simulink model "water_4hopper_VDF"  (Simulink 8.0)
settings: Solver=ode23  StartTime=0.0  StopTime=30  RelTol=1e-3
values from neighbouring files (symbols this model uses):
  alpha = 30    [SimParam_4VDF.m]
  Amp = leg_length    (= 0.0249)    [SimParam_4VDF.m]
  b_water = 0.5*C_d*S1*density    (= 0.405708731037)    [SimParam_4VDF.m]
  C_d = 0.703    [SimParam.m]    (also in SimParam_4VDF.m)
  density = 1000    [SimParam.m]    (also in SimParam_4VDF.m)
  frame_inertia = diag([Ix,Iy,Iz])    [SimParam.m]    (also in SimParam_4VDF.m)
  Fratio = 1/16    (= 0.0625)    [SimParam_4VDF.m]
  freq = 20    [SimParam.m]    (also in SimParam_4VDF.m = 60)
  g = 9.81    [SimParam.m]    (also in SimParam_4VDF.m)
  k_water = C_d*S1*density*g    (= 7.96000530294)    [SimParam_4VDF.m]
  leg_length = 0.06    [SimParam.m]    (also in SimParam_4VDF.m = 0.0249)
  Lx = frame_width/2*[-1 -1 1 1]'    [SimParam_4VDF.m]
  Lxmat = frame_width/2*[-1 0 0 0 ; 0 -1 0 0 ; 0 0 1 0 ; 0 0 0 1]    [SimParam_4VDF.m]
  Lz = frame_length/2*[-1 1 1 -1]'    [SimParam_4VDF.m]
  Lzmat = frame_length/2*[-1 0 0 0 ; 0 1 0 0 ; 0 0 1 0 ; 0 0 0 -1]    [SimParam_4VDF.m]
  mass = 0.1    [SimParam.m]    (also in SimParam_4VDF.m)
  mass_matrix = [mass 0 0; 0 Ix 0 ; 0 0 Iz]    [SimParam_4VDF.m]
  omega_0 = freq*ones(8,1)    [SimParam_4VDF.m]
  S1 = pi*r1^2    (= 0.00125663706144)    [SimParam.m]    (also in SimParam_4VDF.m = 0.00115422114093)
  S2 = pi*r2^2    (= 7.85398163397e-05)    [SimParam.m]    (also in SimParam_4VDF.m = 7.21388213081e-05)
  tau = 0.005    [SimParam_4VDF.m]
  wave = eps    [SimParam_4VDF.m]
  wavefreq = .5    (= 0.5)    [SimParam_4VDF.m]
undefined symbols (not defined in the file): amp, cw_FL_HL, cw_FR_FL, cw_FR_HR, cw_HR_HL, Filter_Coef, FL_HL_lag, FR_FL_lag, FR_HR_lag, HR_HL_lag, K_d, K_i, K_p, y_0
libraries: mblibv1 x34, dspstat3 x6, dspinverses x1
(part 2 of 2)

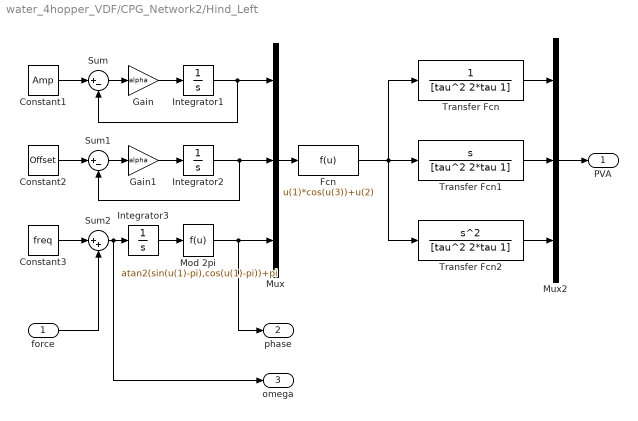
== system water_4hopper_VDF/CPG_Network2/Hind_Left ==
  force : Inport
  Constant1 : Constant  Value=Amp
  Constant2 : Constant  Value=Offset
  Constant3 : Constant  Value=freq
  Fcn : Fcn  Expr=u(1)*cos(u(3))+u(2)
  Gain : Gain  Gain=alpha
  Gain1 : Gain  Gain=alpha
  Integrator1 : Integrator
  Integrator2 : Integrator
  Integrator3 : Integrator  InitialCondition=init_phi + 0.01*rand
  Mod 2pi : Fcn  Expr=atan2(sin(u(1)-pi),cos(u(1)-pi))+pi
  Mux : Mux  Inputs=3
  Mux2 : Mux  Inputs=3
  Sum : Sum  Inputs=|+-
  Sum1 : Sum  Inputs=|+-
  Sum2 : Sum  Inputs=|++
  Transfer Fcn : TransferFcn  Denominator=[tau^2 2*tau 1]
  Transfer Fcn1 : TransferFcn  Numerator=[1 0]  Denominator=[tau^2 2*tau 1]
  Transfer Fcn2 : TransferFcn  Numerator=[1 0 0]  Denominator=[tau^2 2*tau 1]
  PVA : Outport
  phase : Outport  Port=2
  omega : Outport  Port=3
  wires:
  Sum/1 -> Gain/1
  Integrator1/1 -> Sum/2, Mux/1
  Constant1/1 -> Sum/1
  Gain/1 -> Integrator1/1
  Sum1/1 -> Gain1/1
  Integrator2/1 -> Sum1/2, Mux/2
  Constant2/1 -> Sum1/1
  Gain1/1 -> Integrator2/1
  Mux/1 -> Fcn/1
  Mod 2pi/1 -> phase/1, Mux/3
  Integrator3/1 -> Mod 2pi/1
  Constant3/1 -> Sum2/1
  Sum2/1 -> omega/1, Integrator3/1
  force/1 -> Sum2/2
  Transfer Fcn2/1 -> Mux2/3
  Transfer Fcn/1 -> Mux2/1
  Transfer Fcn1/1 -> Mux2/2
  Fcn/1 -> Transfer Fcn2/1, Transfer Fcn/1, Transfer Fcn1/1
  Mux2/1 -> PVA/1

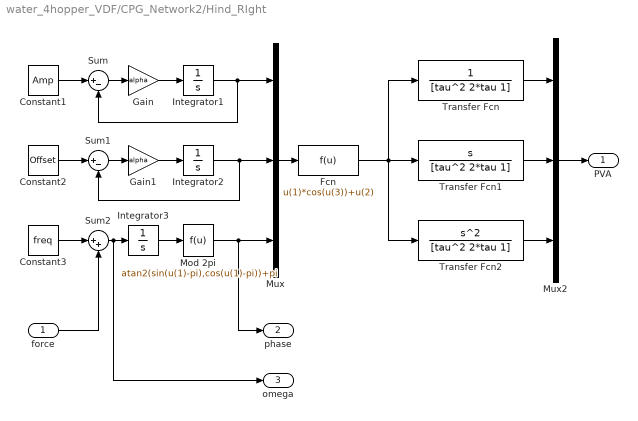
== system water_4hopper_VDF/CPG_Network2/Hind_RIght ==
  force : Inport
  Constant1 : Constant  Value=Amp
  Constant2 : Constant  Value=Offset
  Constant3 : Constant  Value=freq
  Fcn : Fcn  Expr=u(1)*cos(u(3))+u(2)
  Gain : Gain  Gain=alpha
  Gain1 : Gain  Gain=alpha
  Integrator1 : Integrator
  Integrator2 : Integrator
  Integrator3 : Integrator  InitialCondition=init_phi + 0.01*rand
  Mod 2pi : Fcn  Expr=atan2(sin(u(1)-pi),cos(u(1)-pi))+pi
  Mux : Mux  Inputs=3
  Mux2 : Mux  Inputs=3
  Sum : Sum  Inputs=|+-
  Sum1 : Sum  Inputs=|+-
  Sum2 : Sum  Inputs=|++
  Transfer Fcn : TransferFcn  Denominator=[tau^2 2*tau 1]
  Transfer Fcn1 : TransferFcn  Numerator=[1 0]  Denominator=[tau^2 2*tau 1]
  Transfer Fcn2 : TransferFcn  Numerator=[1 0 0]  Denominator=[tau^2 2*tau 1]
  PVA : Outport
  phase : Outport  Port=2
  omega : Outport  Port=3
  wires:
  Sum/1 -> Gain/1
  Integrator1/1 -> Sum/2, Mux/1
  Constant1/1 -> Sum/1
  Gain/1 -> Integrator1/1
  Sum1/1 -> Gain1/1
  Integrator2/1 -> Sum1/2, Mux/2
  Constant2/1 -> Sum1/1
  Gain1/1 -> Integrator2/1
  Mux/1 -> Fcn/1
  Mod 2pi/1 -> phase/1, Mux/3
  Integrator3/1 -> Mod 2pi/1
  Constant3/1 -> Sum2/1
  Sum2/1 -> omega/1, Integrator3/1
  force/1 -> Sum2/2
  Transfer Fcn2/1 -> Mux2/3
  Transfer Fcn/1 -> Mux2/1
  Transfer Fcn1/1 -> Mux2/2
  Fcn/1 -> Transfer Fcn2/1, Transfer Fcn/1, Transfer Fcn1/1
  Mux2/1 -> PVA/1

== system water_4hopper_VDF/CPG_Network2/split FL ==
  w_pos : Inport
  PVA : Inport  Port=2
  w_neg : Inport  Port=3
  Product : Product  RndMeth=Zero
  Product1 : Product  RndMeth=Zero
  Sum2 : Sum  Inputs=|++
  enable : Subsystem
  sel : Selector  InputPortWidth=3  IndexOptions=Index vector (dialog)  Indices=[2]  OutputSizes=1
  Force : Outport
  wires:
  Product/1 -> Sum2/1
  w_pos/1 -> Product/1
  w_neg/1 -> Product1/1
  Product1/1 -> Sum2/2
  PVA/1 -> sel/1
  enable/1(pos) -> Product/2
  enable/2(neg) -> Product1/2
  Sum2/1 -> Force/1
  sel/1 -> enable/1(in)

== system water_4hopper_VDF/CPG_Network2/split FL1 ==
  w_pos : Inport
  PVA : Inport  Port=2
  w_neg : Inport  Port=3
  Product : Product  RndMeth=Zero
  Product1 : Product  RndMeth=Zero
  Sum2 : Sum  Inputs=|++
  enable : Subsystem
  sel : Selector  InputPortWidth=3  IndexOptions=Index vector (dialog)  Indices=[2]  OutputSizes=1
  Force : Outport
  wires:
  sel/1 -> enable/1(in)
  Sum2/1 -> Force/1
  enable/2(neg) -> Product1/2
  enable/1(pos) -> Product/2
  PVA/1 -> sel/1
  Product1/1 -> Sum2/2
  w_neg/1 -> Product1/1
  w_pos/1 -> Product/1
  Product/1 -> Sum2/1

== system water_4hopper_VDF/CPG_Network2/split FL2 ==
  w_pos : Inport
  PVA : Inport  Port=2
  w_neg : Inport  Port=3
  Product : Product  RndMeth=Zero
  Product1 : Product  RndMeth=Zero
  Sum2 : Sum  Inputs=|++
  enable : Subsystem
  sel : Selector  InputPortWidth=3  IndexOptions=Index vector (dialog)  Indices=[2]  OutputSizes=1
  Force : Outport
  wires:
  Product/1 -> Sum2/1
  w_pos/1 -> Product/1
  w_neg/1 -> Product1/1
  Product1/1 -> Sum2/2
  PVA/1 -> sel/1
  enable/1(pos) -> Product/2
  enable/2(neg) -> Product1/2
  Sum2/1 -> Force/1
  sel/1 -> enable/1(in)

== system water_4hopper_VDF/CPG_Network2/split FL3 ==
  w_pos : Inport
  PVA : Inport  Port=2
  w_neg : Inport  Port=3
  Product : Product  RndMeth=Zero
  Product1 : Product  RndMeth=Zero
  Sum2 : Sum  Inputs=|++
  enable : Subsystem
  sel : Selector  InputPortWidth=3  IndexOptions=Index vector (dialog)  Indices=[2]  OutputSizes=1
  Force : Outport
  wires:
  Product/1 -> Sum2/1
  w_pos/1 -> Product/1
  w_neg/1 -> Product1/1
  Product1/1 -> Sum2/2
  PVA/1 -> sel/1
  enable/1(pos) -> Product/2
  enable/2(neg) -> Product1/2
  Sum2/1 -> Force/1
  sel/1 -> enable/1(in)

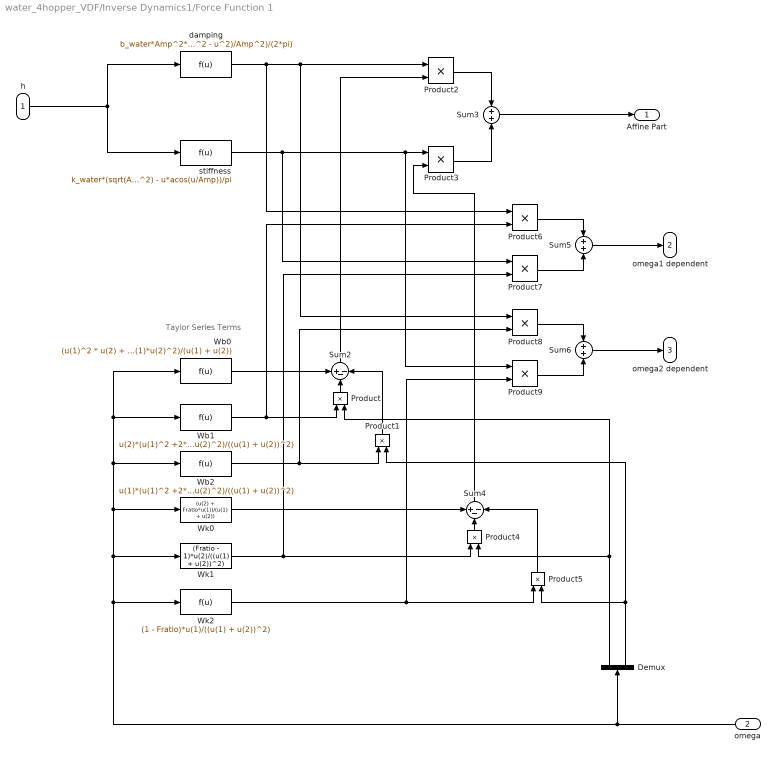
== system water_4hopper_VDF/Inverse Dynamics1/Force Function 1 ==
  note: Taylor Series Terms
  h : Inport
  omega : Inport  Port=2
  Demux : Demux  Outputs=2
  Product{,1..9} (10 alike) : Product  RndMeth=Zero
  Sum2 : Sum  Inputs=+--
  Sum3 : Sum  Inputs=+|+
  Sum4 : Sum  Inputs=+--
  Sum5 : Sum  Inputs=+|+
  Sum6 : Sum  Inputs=+|+
  Wb0 : Fcn  Expr=(u(1)^2 * u(2) + Fratio*u(1)*u(2)^2)/(u(1) + u(2))
  Wb1 : Fcn  Expr=u(2)*(u(1)^2 +2*u(1)*u(2) + Fratio*u(2)^2)/((u(1) + u(2))^2)
  Wb2 : Fcn  Expr=u(1)*(u(1)^2 +2*Fratio*u(1)*u(2) + Fratio*u(2)^2)/((u(1) + u(2))^2)
  Wk0 : Fcn  Expr=(u(2) + Fratio*u(1))/(u(1) + u(2))
  Wk1 : Fcn  Expr=(Fratio - 1)*u(2)/((u(1) + u(2))^2)
  Wk2 : Fcn  Expr=(1 - Fratio)*u(1)/((u(1) + u(2))^2)
  damping : Fcn  Expr=b_water*Amp^2*(acos(u/Amp) - u*sqrt(Amp^2 - u^2)/Amp^2)/(2*pi)
  stiffness : Fcn  Expr=k_water*(sqrt(Amp^2 - u^2) - u*acos(u/Amp))/pi
  Affine Part : Outport
  omega1 dependent : Outport  Port=2
  omega2 dependent : Outport  Port=3
  wires:
  Product2/1 -> Sum3/1
  Product9/1 -> Sum6/2
  Wb1/1 -> Product6/2, Product/1
  Product4/1 -> Sum4/2
  Wb0/1 -> Sum2/1
  Product7/1 -> Sum5/2
  Wk1/1 -> Product7/2, Product4/1
  Wk0/1 -> Sum4/1
  Product6/1 -> Sum5/1
  Wb2/1 -> Product8/2, Product1/1
  Product/1 -> Sum2/2
  Sum3/1 -> Affine Part/1
  Product1/1 -> Sum2/3
  stiffness/1 -> Product7/1, Product9/1, Product3/1
  Wk2/1 -> Product5/1, Product9/2
  damping/1 -> Product6/1, Product8/1, Product2/1
  Product5/1 -> Sum4/3
  Product3/1 -> Sum3/2
  Sum5/1 -> omega1 dependent/1
  Sum4/1 -> Product3/2
  omega/1 -> Wb0/1, Wb1/1, Wb2/1, Wk0/1, Wk1/1, Wk2/1, Demux/1
  Sum2/1 -> Product2/2
  Product8/1 -> Sum6/1
  Sum6/1 -> omega2 dependent/1
  Demux/1 -> Product4/2, Product/2
  Demux/2 -> Product5/2, Product1/2
  h/1 -> stiffness/1, damping/1

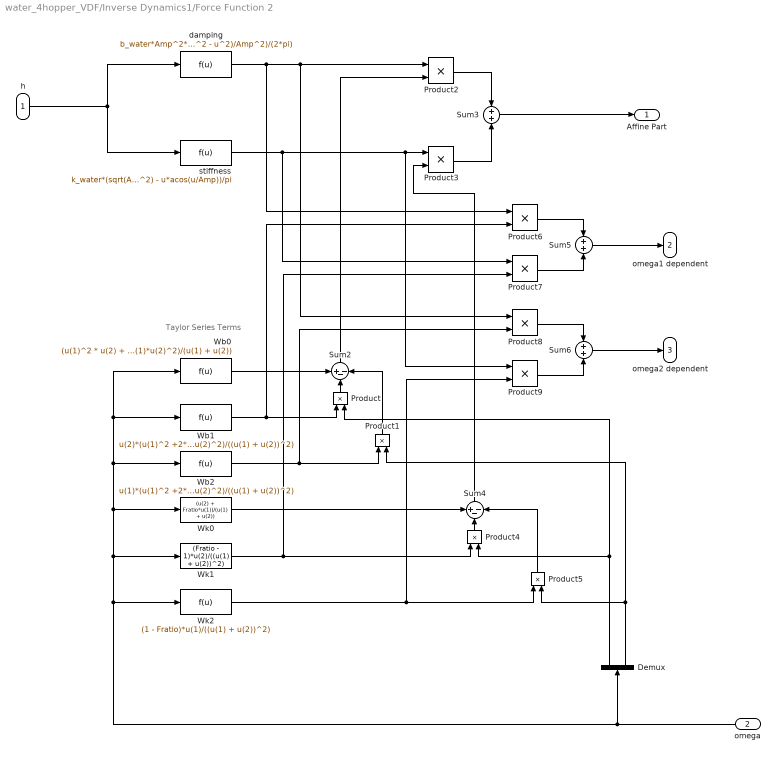
== system water_4hopper_VDF/Inverse Dynamics1/Force Function 2 ==
  note: Taylor Series Terms
  h : Inport
  omega : Inport  Port=2
  Demux : Demux  Outputs=2
  Product{,1..9} (10 alike) : Product  RndMeth=Zero
  Sum2 : Sum  Inputs=+--
  Sum3 : Sum  Inputs=+|+
  Sum4 : Sum  Inputs=+--
  Sum5 : Sum  Inputs=+|+
  Sum6 : Sum  Inputs=+|+
  Wb0 : Fcn  Expr=(u(1)^2 * u(2) + Fratio*u(1)*u(2)^2)/(u(1) + u(2))
  Wb1 : Fcn  Expr=u(2)*(u(1)^2 +2*u(1)*u(2) + Fratio*u(2)^2)/((u(1) + u(2))^2)
  Wb2 : Fcn  Expr=u(1)*(u(1)^2 +2*Fratio*u(1)*u(2) + Fratio*u(2)^2)/((u(1) + u(2))^2)
  Wk0 : Fcn  Expr=(u(2) + Fratio*u(1))/(u(1) + u(2))
  Wk1 : Fcn  Expr=(Fratio - 1)*u(2)/((u(1) + u(2))^2)
  Wk2 : Fcn  Expr=(1 - Fratio)*u(1)/((u(1) + u(2))^2)
  damping : Fcn  Expr=b_water*Amp^2*(acos(u/Amp) - u*sqrt(Amp^2 - u^2)/Amp^2)/(2*pi)
  stiffness : Fcn  Expr=k_water*(sqrt(Amp^2 - u^2) - u*acos(u/Amp))/pi
  Affine Part : Outport
  omega1 dependent : Outport  Port=2
  omega2 dependent : Outport  Port=3
  wires:
  Product2/1 -> Sum3/1
  Product9/1 -> Sum6/2
  Wb1/1 -> Product6/2, Product/1
  Product4/1 -> Sum4/2
  Wb0/1 -> Sum2/1
  Product7/1 -> Sum5/2
  Wk1/1 -> Product7/2, Product4/1
  Wk0/1 -> Sum4/1
  Product6/1 -> Sum5/1
  Wb2/1 -> Product8/2, Product1/1
  Product/1 -> Sum2/2
  Sum3/1 -> Affine Part/1
  Product1/1 -> Sum2/3
  stiffness/1 -> Product7/1, Product9/1, Product3/1
  Wk2/1 -> Product5/1, Product9/2
  damping/1 -> Product6/1, Product8/1, Product2/1
  Product5/1 -> Sum4/3
  Product3/1 -> Sum3/2
  Sum5/1 -> omega1 dependent/1
  Sum4/1 -> Product3/2
  omega/1 -> Wb0/1, Wb1/1, Wb2/1, Wk0/1, Wk1/1, Wk2/1, Demux/1
  Sum2/1 -> Product2/2
  Product8/1 -> Sum6/1
  Sum6/1 -> omega2 dependent/1
  Demux/1 -> Product4/2, Product/2
  Demux/2 -> Product5/2, Product1/2
  h/1 -> stiffness/1, damping/1

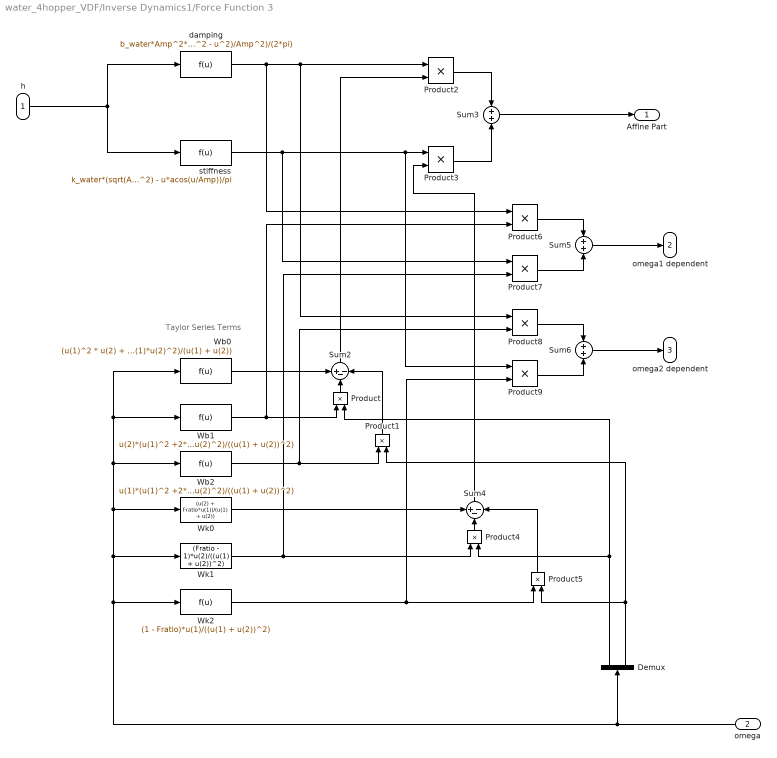
== system water_4hopper_VDF/Inverse Dynamics1/Force Function 3 ==
  note: Taylor Series Terms
  h : Inport
  omega : Inport  Port=2
  Demux : Demux  Outputs=2
  Product{,1..9} (10 alike) : Product  RndMeth=Zero
  Sum2 : Sum  Inputs=+--
  Sum3 : Sum  Inputs=+|+
  Sum4 : Sum  Inputs=+--
  Sum5 : Sum  Inputs=+|+
  Sum6 : Sum  Inputs=+|+
  Wb0 : Fcn  Expr=(u(1)^2 * u(2) + Fratio*u(1)*u(2)^2)/(u(1) + u(2))
  Wb1 : Fcn  Expr=u(2)*(u(1)^2 +2*u(1)*u(2) + Fratio*u(2)^2)/((u(1) + u(2))^2)
  Wb2 : Fcn  Expr=u(1)*(u(1)^2 +2*Fratio*u(1)*u(2) + Fratio*u(2)^2)/((u(1) + u(2))^2)
  Wk0 : Fcn  Expr=(u(2) + Fratio*u(1))/(u(1) + u(2))
  Wk1 : Fcn  Expr=(Fratio - 1)*u(2)/((u(1) + u(2))^2)
  Wk2 : Fcn  Expr=(1 - Fratio)*u(1)/((u(1) + u(2))^2)
  damping : Fcn  Expr=b_water*Amp^2*(acos(u/Amp) - u*sqrt(Amp^2 - u^2)/Amp^2)/(2*pi)
  stiffness : Fcn  Expr=k_water*(sqrt(Amp^2 - u^2) - u*acos(u/Amp))/pi
  Affine Part : Outport
  omega1 dependent : Outport  Port=2
  omega2 dependent : Outport  Port=3
  wires:
  Product2/1 -> Sum3/1
  Product9/1 -> Sum6/2
  Wb1/1 -> Product6/2, Product/1
  Product4/1 -> Sum4/2
  Wb0/1 -> Sum2/1
  Product7/1 -> Sum5/2
  Wk1/1 -> Product7/2, Product4/1
  Wk0/1 -> Sum4/1
  Product6/1 -> Sum5/1
  Wb2/1 -> Product8/2, Product1/1
  Product/1 -> Sum2/2
  Sum3/1 -> Affine Part/1
  Product1/1 -> Sum2/3
  stiffness/1 -> Product7/1, Product9/1, Product3/1
  Wk2/1 -> Product5/1, Product9/2
  damping/1 -> Product6/1, Product8/1, Product2/1
  Product5/1 -> Sum4/3
  Product3/1 -> Sum3/2
  Sum5/1 -> omega1 dependent/1
  Sum4/1 -> Product3/2
  omega/1 -> Wb0/1, Wb1/1, Wb2/1, Wk0/1, Wk1/1, Wk2/1, Demux/1
  Sum2/1 -> Product2/2
  Product8/1 -> Sum6/1
  Sum6/1 -> omega2 dependent/1
  Demux/1 -> Product4/2, Product/2
  Demux/2 -> Product5/2, Product1/2
  h/1 -> stiffness/1, damping/1

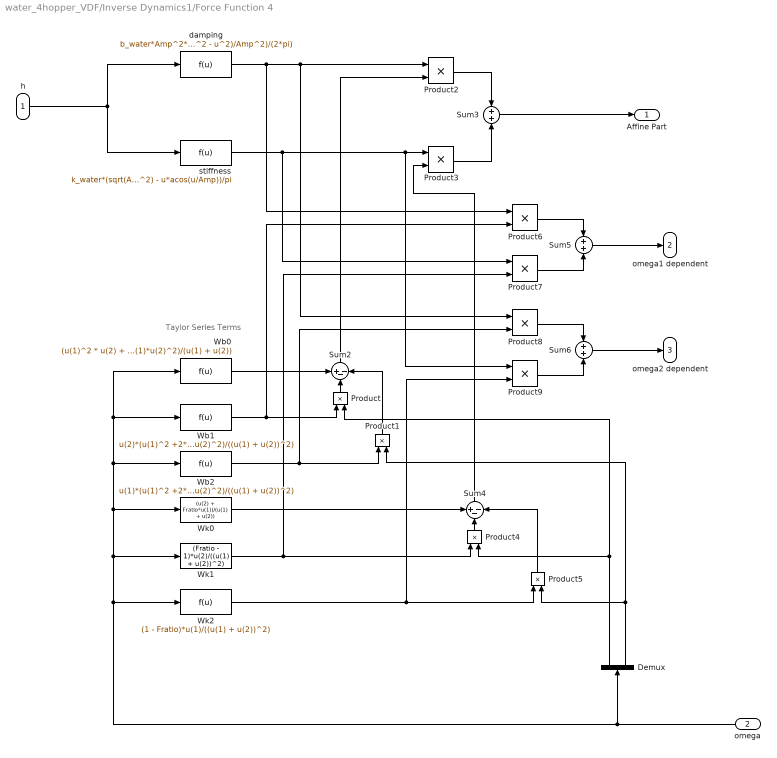
== system water_4hopper_VDF/Inverse Dynamics1/Force Function 4 ==
  note: Taylor Series Terms
  h : Inport
  omega : Inport  Port=2
  Demux : Demux  Outputs=2
  Product{,1..9} (10 alike) : Product  RndMeth=Zero
  Sum2 : Sum  Inputs=+--
  Sum3 : Sum  Inputs=+|+
  Sum4 : Sum  Inputs=+--
  Sum5 : Sum  Inputs=+|+
  Sum6 : Sum  Inputs=+|+
  Wb0 : Fcn  Expr=(u(1)^2 * u(2) + Fratio*u(1)*u(2)^2)/(u(1) + u(2))
  Wb1 : Fcn  Expr=u(2)*(u(1)^2 +2*u(1)*u(2) + Fratio*u(2)^2)/((u(1) + u(2))^2)
  Wb2 : Fcn  Expr=u(1)*(u(1)^2 +2*Fratio*u(1)*u(2) + Fratio*u(2)^2)/((u(1) + u(2))^2)
  Wk0 : Fcn  Expr=(u(2) + Fratio*u(1))/(u(1) + u(2))
  Wk1 : Fcn  Expr=(Fratio - 1)*u(2)/((u(1) + u(2))^2)
  Wk2 : Fcn  Expr=(1 - Fratio)*u(1)/((u(1) + u(2))^2)
  damping : Fcn  Expr=b_water*Amp^2*(acos(u/Amp) - u*sqrt(Amp^2 - u^2)/Amp^2)/(2*pi)
  stiffness : Fcn  Expr=k_water*(sqrt(Amp^2 - u^2) - u*acos(u/Amp))/pi
  Affine Part : Outport
  omega1 dependent : Outport  Port=2
  omega2 dependent : Outport  Port=3
  wires:
  Product2/1 -> Sum3/1
  Product9/1 -> Sum6/2
  Wb1/1 -> Product6/2, Product/1
  Product4/1 -> Sum4/2
  Wb0/1 -> Sum2/1
  Product7/1 -> Sum5/2
  Wk1/1 -> Product7/2, Product4/1
  Wk0/1 -> Sum4/1
  Product6/1 -> Sum5/1
  Wb2/1 -> Product8/2, Product1/1
  Product/1 -> Sum2/2
  Sum3/1 -> Affine Part/1
  Product1/1 -> Sum2/3
  stiffness/1 -> Product7/1, Product9/1, Product3/1
  Wk2/1 -> Product5/1, Product9/2
  damping/1 -> Product6/1, Product8/1, Product2/1
  Product5/1 -> Sum4/3
  Product3/1 -> Sum3/2
  Sum5/1 -> omega1 dependent/1
  Sum4/1 -> Product3/2
  omega/1 -> Wb0/1, Wb1/1, Wb2/1, Wk0/1, Wk1/1, Wk2/1, Demux/1
  Sum2/1 -> Product2/2
  Product8/1 -> Sum6/1
  Sum6/1 -> omega2 dependent/1
  Demux/1 -> Product4/2, Product/2
  Demux/2 -> Product5/2, Product1/2
  h/1 -> stiffness/1, damping/1

== system water_4hopper_VDF/Inverse Dynamics1/PID ==
  In1 : Inport
  Derivative Gain : Gain  Gain=D  Multiplication=Matrix(K*u)
  Gain : Gain  Gain=N
  Integral Gain : Gain  DisableCoverage=on  Gain=I  Multiplication=Matrix(K*u)
  Integrator : Integrator
  Integrator1 : Integrator
  Proportional Gain : Gain  Gain=P  Multiplication=Matrix(K*u)
  Sum : Sum  Inputs=|+-
  Sum11 : Sum  Inputs=+++
  Out1 : Outport
  wires:
  Proportional Gain/1 -> Sum11/1
  Integral Gain/1 -> Integrator/1
  Sum11/1 -> Out1/1
  Integrator/1 -> Sum11/2
  In1/1 -> Derivative Gain/1, Integral Gain/1, Proportional Gain/1
  Gain/1 -> Sum11/3, Integrator1/1
  Sum/1 -> Gain/1
  Integrator1/1 -> Sum/2
  Derivative Gain/1 -> Sum/1

== system water_4hopper_VDF/leg L1/Subsystem ==
  pos : Inport
  vel : Inport  Port=2
  Constant : Constant  Value=0
  Gain : Gain  Gain=C_d*density
  Gain1 : Gain  Gain=-0.5
  Gain2 : Gain  Gain=S1
  Gain3 : Gain  Gain=g
  Gain4 : Gain  Gain=S2
  Gain5 : Gain  Gain=0.5
  Math Function : Math  Operator=square  SaturateOnIntegerOverflow=on
  Sum : Sum  Inputs=-+|
  Sum1 : Sum  Inputs=-+|
  Switch : Switch  ZeroCross=off
  Switch1 : Switch
  force : Outport
  wires:
  vel/1 -> Switch/2, Math Function/1
  Math Function/1 -> Gain1/1, Gain5/1
  Gain1/1 -> Sum/2
  pos/1 -> Gain3/1, Switch1/2
  Gain3/1 -> Sum/1, Sum1/1
  Sum/1 -> Gain4/1
  Gain4/1 -> Switch/1
  Gain2/1 -> Switch/3
  Switch/1 -> Gain/1
  Switch1/1 -> force/1
  Gain/1 -> Switch1/3
  Constant/1 -> Switch1/1
  Sum1/1 -> Gain2/1
  Gain5/1 -> Sum1/2

== system water_4hopper_VDF/leg L2/Subsystem ==
  pos : Inport
  vel : Inport  Port=2
  Constant : Constant  Value=0
  Gain : Gain  Gain=C_d*density
  Gain1 : Gain  Gain=-0.5
  Gain2 : Gain  Gain=S1
  Gain3 : Gain  Gain=g
  Gain4 : Gain  Gain=S2
  Gain5 : Gain  Gain=0.5
  Math Function : Math  Operator=square  SaturateOnIntegerOverflow=on
  Sum : Sum  Inputs=-+|
  Sum1 : Sum  Inputs=-+|
  Switch : Switch  ZeroCross=off
  Switch1 : Switch
  force : Outport
  wires:
  vel/1 -> Switch/2, Math Function/1
  Math Function/1 -> Gain1/1, Gain5/1
  Gain1/1 -> Sum/2
  pos/1 -> Gain3/1, Switch1/2
  Gain3/1 -> Sum/1, Sum1/1
  Sum/1 -> Gain4/1
  Gain4/1 -> Switch/1
  Gain2/1 -> Switch/3
  Switch/1 -> Gain/1
  Switch1/1 -> force/1
  Gain/1 -> Switch1/3
  Constant/1 -> Switch1/1
  Sum1/1 -> Gain2/1
  Gain5/1 -> Sum1/2

== system water_4hopper_VDF/leg L3/Subsystem ==
  pos : Inport
  vel : Inport  Port=2
  Constant : Constant  Value=0
  Gain : Gain  Gain=C_d*density
  Gain1 : Gain  Gain=-0.5
  Gain2 : Gain  Gain=S1
  Gain3 : Gain  Gain=g
  Gain4 : Gain  Gain=S2
  Gain5 : Gain  Gain=0.5
  Math Function : Math  Operator=square  SaturateOnIntegerOverflow=on
  Sum : Sum  Inputs=-+|
  Sum1 : Sum  Inputs=-+|
  Switch : Switch  ZeroCross=off
  Switch1 : Switch
  force : Outport
  wires:
  vel/1 -> Switch/2, Math Function/1
  Math Function/1 -> Gain1/1, Gain5/1
  Gain1/1 -> Sum/2
  pos/1 -> Gain3/1, Switch1/2
  Gain3/1 -> Sum/1, Sum1/1
  Sum/1 -> Gain4/1
  Gain4/1 -> Switch/1
  Gain2/1 -> Switch/3
  Switch/1 -> Gain/1
  Switch1/1 -> force/1
  Gain/1 -> Switch1/3
  Constant/1 -> Switch1/1
  Sum1/1 -> Gain2/1
  Gain5/1 -> Sum1/2

== system water_4hopper_VDF/leg L4/Subsystem ==
  pos : Inport
  vel : Inport  Port=2
  Constant : Constant  Value=0
  Gain : Gain  Gain=C_d*density
  Gain1 : Gain  Gain=-0.5
  Gain2 : Gain  Gain=S1
  Gain3 : Gain  Gain=g
  Gain4 : Gain  Gain=S2
  Gain5 : Gain  Gain=0.5
  Math Function : Math  Operator=square  SaturateOnIntegerOverflow=on
  Sum : Sum  Inputs=-+|
  Sum1 : Sum  Inputs=-+|
  Switch : Switch  ZeroCross=off
  Switch1 : Switch
  force : Outport
  wires:
  vel/1 -> Switch/2, Math Function/1
  Math Function/1 -> Gain1/1, Gain5/1
  Gain1/1 -> Sum/2
  pos/1 -> Gain3/1, Switch1/2
  Gain3/1 -> Sum/1, Sum1/1
  Sum/1 -> Gain4/1
  Gain4/1 -> Switch/1
  Gain2/1 -> Switch/3
  Switch/1 -> Gain/1
  Switch1/1 -> force/1
  Gain/1 -> Switch1/3
  Constant/1 -> Switch1/1
  Sum1/1 -> Gain2/1
  Gain5/1 -> Sum1/2

== system water_4hopper_VDF/CPG_Network2/split FL/enable ==
  in : Inport
  Constant1 : Constant
  Constant2 : Constant
  Derivative : Derivative
  Gain : Gain  Gain=.5
  Gain1 : Gain  Gain=.5
  Sign : Signum
  Sum1 : Sum  Inputs=|++
  Sum2 : Sum  Inputs=|-+
  pos : Outport
  neg : Outport  Port=2
  wires:
  Derivative/1 -> Sign/1
  Constant1/1 -> Sum1/2
  Sign/1 -> Sum2/1, Sum1/1
  Gain/1 -> pos/1
  in/1 -> Derivative/1
  Sum1/1 -> Gain/1
  Constant2/1 -> Sum2/2
  Gain1/1 -> neg/1
  Sum2/1 -> Gain1/1

== system water_4hopper_VDF/CPG_Network2/split FL1/enable ==
  in : Inport
  Constant1 : Constant
  Constant2 : Constant
  Derivative : Derivative
  Gain : Gain  Gain=.5
  Gain1 : Gain  Gain=.5
  Sign : Signum
  Sum1 : Sum  Inputs=|++
  Sum2 : Sum  Inputs=|-+
  pos : Outport
  neg : Outport  Port=2
  wires:
  Sum2/1 -> Gain1/1
  Gain1/1 -> neg/1
  Constant2/1 -> Sum2/2
  Sum1/1 -> Gain/1
  in/1 -> Derivative/1
  Gain/1 -> pos/1
  Sign/1 -> Sum1/1, Sum2/1
  Constant1/1 -> Sum1/2
  Derivative/1 -> Sign/1

== system water_4hopper_VDF/CPG_Network2/split FL2/enable ==
  in : Inport
  Constant1 : Constant
  Constant2 : Constant
  Derivative : Derivative
  Gain : Gain  Gain=.5
  Gain1 : Gain  Gain=.5
  Sign : Signum
  Sum1 : Sum  Inputs=|++
  Sum2 : Sum  Inputs=|-+
  pos : Outport
  neg : Outport  Port=2
  wires:
  Derivative/1 -> Sign/1
  Constant1/1 -> Sum1/2
  Sign/1 -> Sum2/1, Sum1/1
  Gain/1 -> pos/1
  in/1 -> Derivative/1
  Sum1/1 -> Gain/1
  Constant2/1 -> Sum2/2
  Gain1/1 -> neg/1
  Sum2/1 -> Gain1/1

== system water_4hopper_VDF/CPG_Network2/split FL3/enable ==
  in : Inport
  Constant1 : Constant
  Constant2 : Constant
  Derivative : Derivative
  Gain : Gain  Gain=.5
  Gain1 : Gain  Gain=.5
  Sign : Signum
  Sum1 : Sum  Inputs=|++
  Sum2 : Sum  Inputs=|-+
  pos : Outport
  neg : Outport  Port=2
  wires:
  Derivative/1 -> Sign/1
  Constant1/1 -> Sum1/2
  Sign/1 -> Sum2/1, Sum1/1
  Gain/1 -> pos/1
  in/1 -> Derivative/1
  Sum1/1 -> Gain/1
  Constant2/1 -> Sum2/2
  Gain1/1 -> neg/1
  Sum2/1 -> Gain1/1
